simulink model "sim_act1"  (R2021a)
settings: Solver=VariableStepAuto  StartTime=0.0  StopTime=1  RelTol=1e-3
settings Model: Creator=pierr  LastModifiedBy=pierr

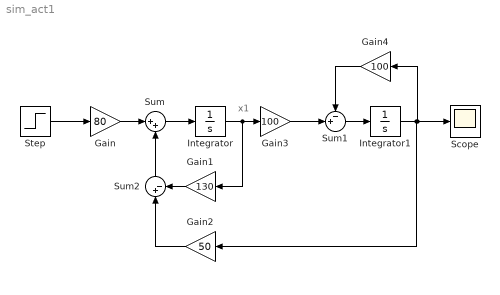
== system sim_act1 ==
  note: x1
  Gain : Gain  Gain=80
  Gain1 : Gain  Gain=130
  Gain2 : Gain  Gain=50
  Gain3 : Gain  Gain=100
  Gain4 : Gain  Gain=100
  Integrator : Integrator
  Integrator1 : Integrator
  Scope : Scope
  Step : Step  Time=0  SampleTime=0
  Sum : Sum  Inputs=|++
  Sum1 : Sum  Inputs=-+|
  Sum2 : Sum  Inputs=|+-
  wires:
  Gain/1 -> Sum/1
  Gain1/1 -> Sum2/2
  Sum/1 -> Integrator/1
  Integrator/1 -> Gain1/1, Gain3/1
  Gain2/1 -> Sum2/1
  Sum2/1 -> Sum/2
  Gain3/1 -> Sum1/2
  Gain4/1 -> Sum1/1
  Sum1/1 -> Integrator1/1
  Integrator1/1 -> Gain2/1, Scope/1, Gain4/1
  Step/1 -> Gain/1
